simulink model "EmbeddedOpenLoop"  (Simulink 10.0)
settings: Solver=ode3  StartTime=0.0  StopTime=10.0  RelTol=1e-3
libraries: arduinolib x5, simulink x2
settings Model: Creator=pvinnako  LastModifiedBy=bhisma  ExtModeTrigDuration=2
settings DataIOCC: LimitDataPoints=on  SignalLoggingSaveFormat=ModelDataLogs
settings OptimizationCC: ExpressionDepthLimit=2147483647  LifeSpan=1  EfficientTunableParamExpr=on
settings DebuggingCC: FcnCallInpInsideContextMsg=warning  StateNameClashWarn=warning
settings HardwareCC: ProdBitPerInt=16  ProdBitPerPointer=16  ProdBitPerSizeT=16  ProdBitPerPtrDiffT=16  ProdIntDivRoundTo=Zero  ProdEndianess=LittleEndian  ProdWordSize=8  ProdHWDeviceType=Atmel->AVR
settings SFSimCC: MATLABDynamicMemAlloc=off
settings RTWCC: Description=Real-Time Toolbox  SystemTargetFile=realtime.tlc  GenerateMakefile=off  TemplateMakefile=realtime.tmf  RTWVerbose=off
settings CodeAppCC: CustomSymbolStrType=$N$R$M  InternalIdentifier=Classic
settings STFCustomTargetCC: TargetLibSuffix=.a  GenerateSampleERTMain=on  ERTCustomFileBanners=on  SupportNonInlinedSFcns=off  RemoveResetFunc=on  SupportVariableSizeSignals=on  MATLABClassNameForMDSCustomization=Simulink.SoftwareTarget.ERTCustomization  GRTInterface=off  SystemTargetFile=realtime.tlc
settings ERTTargetCC: MultiwordLength=2048  GenerateSampleERTMain=on  ParMdlRefBuildCompliant=off  CompOptLevelCompliant=off  ConcurrentExecutionCompliant=off  CombineOutputUpdateFcns=off  SupportContinuousTime=on  SupportVariableSizeSignals=on  ModelStepFunctionPrototypeControlCompliant=off  CPPClassGenCompliant=off  UseToolchainInfoCompliant=off  ExtModeTransport=3  ExtModeMexFile=ext_serial_win32_comm  ExtModeMexArgs=0 1 9600  ERTSrcFileBannerTemplate=realtime_code_template.cgt  ERTHdrFileBannerTemplate=realtime_code_template.cgt  ERTDataSrcFileTemplate=realtime_code_template.cgt  ERTDataHdrFileTemplate=realtime_code_template.cgt  ERTCustomFileTemplate=realtime_file_process.tlc  ConvertIfToSwitch=off  SuppressUnreachableDefaultCases=off
settings ConfigComp: CovExternalEMLEnable=off
settings SettingsController: Description=Run on Hardware Dialog  TargetExtensionPlatform=Arduino Uno
settings MATStruct: Set_host_COM_port=[0.0]  COM_port_number=1  COM_port_baud_rate=115200  Enable_overrun_detection=[0.0]  Digital_output_to_set_on_overrun=13  Analog_input_reference_voltage=[0.0]  Serial0_baud_rate=9600

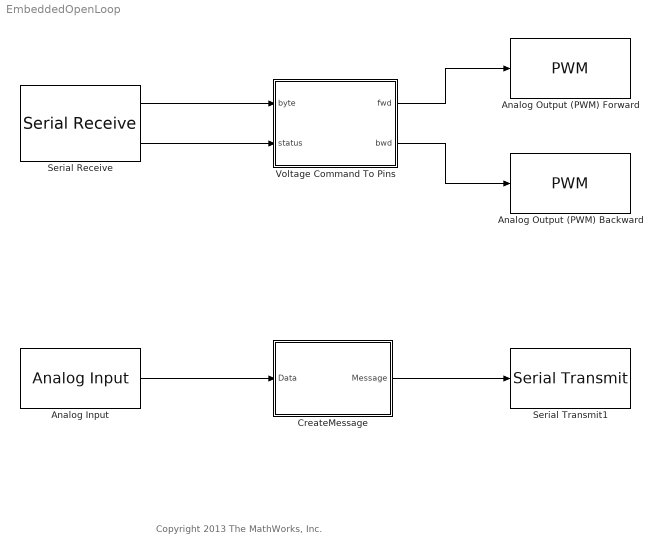
== system EmbeddedOpenLoop ==
  note: Copyright 2013 The MathWorks, Inc.
  Analog Input : arduinolib/Analog Input  pinNumber=0  sampleTime=0.01
  Analog Output (PWM) Backward : arduinolib/PWM  pinNumber=11
  Analog Output (PWM) Forward : arduinolib/PWM  pinNumber=10
  CreateMessage : Subsystem
  Serial Receive : arduinolib/Serial Receive  portNumber=0  showOutStatus=on  sampleTime=0.01
      settings: SourceProductName=Simulink Support Package for Arduino Hardware  SourceProductBaseCode=ARDUINO
  Serial Transmit1 : arduinolib/Serial Transmit  portNumber=0
      settings: SourceProductName=Simulink Support Package for Arduino Hardware
  Voltage Command To Pins : MATLAB Function  TreatAsAtomicUnit=on
  wires:
  Voltage Command To Pins/1(fwd) -> Analog Output (PWM) Forward/1
  Analog Input/1 -> CreateMessage/1(Data)
  Serial Receive/1 -> Voltage Command To Pins/1(byte)
  CreateMessage/1(Message) -> Serial Transmit1/1
  Serial Receive/2 -> Voltage Command To Pins/2(status)
  Voltage Command To Pins/2(bwd) -> Analog Output (PWM) Backward/1

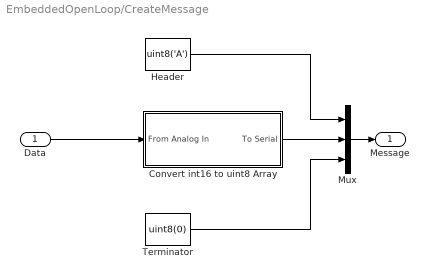
== system EmbeddedOpenLoop/CreateMessage ==
  Data : Inport
  Convert int16 to uint8 Array : Subsystem
  Header : Constant  Value=uint8('A')
  Mux : Mux  Inputs=3
  Terminator : Constant  Value=uint8(0)
  Message : Outport
  wires:
  Header/1 -> Mux/1
  Terminator/1 -> Mux/3
  Data/1 -> Convert int16 to uint8 Array/1(From Analog In)
  Mux/1 -> Message/1
  Convert int16 to uint8 Array/1(To Serial) -> Mux/2

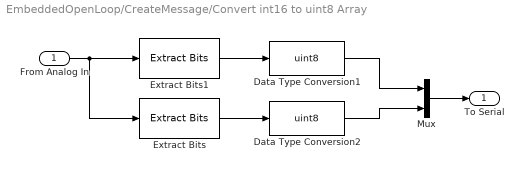
== system EmbeddedOpenLoop/CreateMessage/Convert int16 to uint8 Array ==
  From Analog In : Inport
  Data Type Conversion1 : DataTypeConversion  OutDataTypeStr=uint8  ConvertRealWorld=Stored Integer (SI)
  Data Type Conversion2 : DataTypeConversion  OutDataTypeStr=uint8  ConvertRealWorld=Stored Integer (SI)
  Extract Bits : simulink/Logic and Bit Operations/Extract Bits  bitsToExtract=Upper half  numBits=8  bitIdxRange=[0 7]  outScalingMode=Treat bit field as an integer
      settings: SourceProductName=Simulink
  Extract Bits1 : simulink/Logic and Bit Operations/Extract Bits  bitsToExtract=Lower half  numBits=8  bitIdxRange=[0 7]  outScalingMode=Treat bit field as an integer
      settings: SourceProductName=Simulink
  Mux : Mux  Inputs=2
  To Serial : Outport
  wires:
  Extract Bits/1 -> Data Type Conversion2/1
  Extract Bits1/1 -> Data Type Conversion1/1
  From Analog In/1 -> Extract Bits1/1, Extract Bits/1
  Mux/1 -> To Serial/1
  Data Type Conversion1/1 -> Mux/1
  Data Type Conversion2/1 -> Mux/2

== matlab function Voltage Command To Pins ==
  data: byte input double; fwd output double; bwd output double; status input double
function [fwd,bwd] = passVolts(byte,status)
%#codegen
persistent last

if isempty(last)
    last = int16(0);
end

if (byte>=0 && status == 1)
    volt = 2*(int16(byte)-127);
    last = volt;
else
    volt = last;
end

if volt>0
    fwd = uint8(volt);
    bwd = uint8(0);
else
    fwd = uint8(0);
    bwd = uint8(-volt);
end
